simulink model "untitled2"  (R2017a)
settings: Solver=VariableStepAuto  StartTime=0.0  StopTime=10.0  RelTol=1e-3
settings Model: Creator=ishaf  LastModifiedBy=sidharth

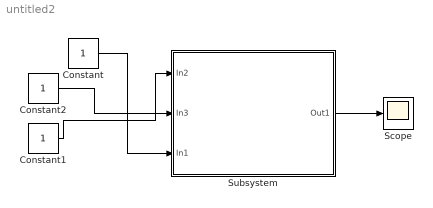
== system untitled2 ==
  Constant : Constant
  Constant1 : Constant
  Constant2 : Constant
  Scope : Scope
  Subsystem : Subsystem
  wires:
  Constant/1 -> Subsystem/3(In1)
  Subsystem/1(Out1) -> Scope/1
  Constant1/1 -> Subsystem/1(In2)
  Constant2/1 -> Subsystem/2(In3)

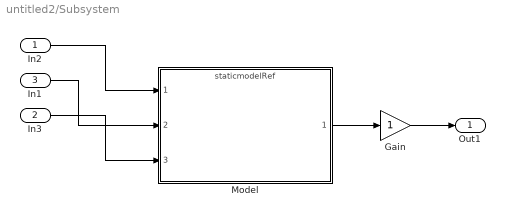
== system untitled2/Subsystem ==
  In2 : Inport
  In3 : Inport  Port=2
  In1 : Inport  Port=3
  Gain : Gain
  Model : ModelReference  ModelNameDialog=staticmodelRef.slx  SimulationMode=Normal  ModelReferenceVersion=1.12
  Out1 : Outport
  wires:
  Gain/1 -> Out1/1
  Model/1 -> Gain/1
  In2/1 -> Model/1
  In1/1 -> Model/2
  In3/1 -> Model/3
